simulink model "kh4_controller_v2"  (R2020a)
settings: Solver=ode15s  StartTime=0.0  StopTime=Inf  RelTol=1e-3
undefined symbols (not defined in the file or in its folder): Angular, Linear
libraries: robotlib x3, simulink x2, dspinverses x1
settings Model: Creator=FlightControlLab  LastModifiedBy=javier
settings SolverCC: SolverResetMethod=Robust
settings DataIOCC: ReturnWorkspaceOutputs=off
settings DebuggingCC: ArithmeticOperatorsInVariantConditions=warning
settings SFSimCC: SimUseLocalCustomCode=off  CustomCodeUndefinedFunction=UseInterfaceOnly
settings RTWCC: RTWUseLocalCustomCode=off

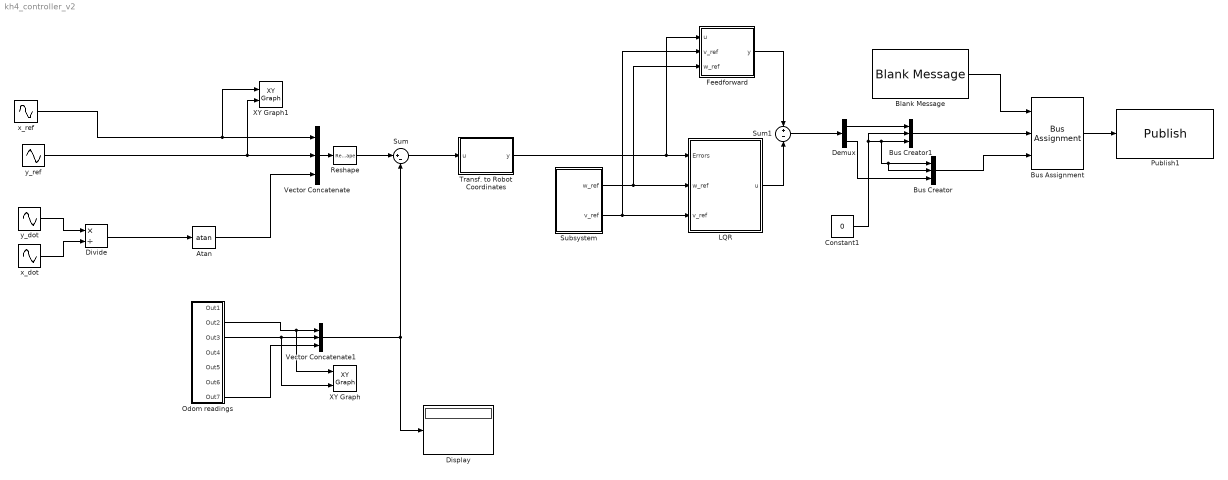
== system kh4_controller_v2 ==
  Atan : Trigonometry  Operator=atan
  Blank Message : robotlib/Blank Message  messageClass=Message  entityType=geometry_msgs/Twist  messageType=geometry_msgs/Twist  SampleTime=inf
  Bus Assignment : BusAssignment  AssignedSignals=Linear,Angular
  Bus Creator : BusCreator  Inputs=3
  Bus Creator1 : BusCreator  Inputs=3
  Constant1 : Constant  Value=0
  Demux : Demux  Outputs=2
  Display : Display
  Divide : Product  Inputs=*/
  Feedforward : MATLAB Function  TreatAsAtomicUnit=on
  LQR : Subsystem
  Odom readings : Subsystem
  Publish1 : robotlib/Publish  topicSource=Select from ROS network  topic=/kh4_diff_drive_controller/cmd_vel  messageType=geometry_msgs/Twist  messageQueueLength=105
  Reshape : Reshape  OutputDimensionality=Column vector (2-D)
  Subsystem : Subsystem
  Sum : Sum  Inputs=|+-
  Sum1 : Sum  Inputs=+-
  Transf. to Robot Coordinates : MATLAB Function  TreatAsAtomicUnit=on
  Vector Concatenate : Concatenate  NumInputs=3
  Vector Concatenate1 : Concatenate  NumInputs=3
  XY Graph : simulink/Sinks/XY Graph  xmin=-1  xmax=1  ymin=-1  ymax=1  st=-1
  XY Graph1 : simulink/Sinks/XY Graph  xmin=-1  xmax=1  ymin=-1  ymax=1  st=-1
  x_dot : Sin  Amplitude=0.3^2  Frequency=0.3  Phase=pi/2  SampleTime=0
  x_ref : Sin  Amplitude=0.3  Frequency=0.3  SampleTime=0
  y_dot : Sin  Amplitude=-0.3^2  Frequency=0.3  SampleTime=0
  y_ref : Sin  Amplitude=0.3  Bias=-0.3  Frequency=0.3  Phase=pi/2  SampleTime=0
  wires:
  x_dot/1 -> Divide/2
  Divide/1 -> Atan/1
  Sum/1 -> Transf. to Robot Coordinates/1(u)
  x_ref/1 -> XY Graph1/1, Vector Concatenate/1
  Vector Concatenate/1 -> Reshape/1
  y_ref/1 -> XY Graph1/2, Vector Concatenate/2
  Reshape/1 -> Sum/1
  Atan/1 -> Vector Concatenate/3
  Transf. to Robot Coordinates/1(y) -> LQR/1(Errors), Feedforward/1(u)
  Feedforward/1(y) -> Sum1/1
  Subsystem/2(v_ref) -> LQR/3(v_ref), Feedforward/2(v_ref)
  y_dot/1 -> Divide/1
  LQR/1(u) -> Sum1/2
  Subsystem/1(w_ref) -> LQR/2(w_ref), Feedforward/3(w_ref)
  Sum1/1 -> Demux/1
  Blank Message/1 -> Bus Assignment/1
  Bus Assignment/1 -> Publish1/1
  Constant1/1 -> Bus Creator1/2, Bus Creator/2, Bus Creator/1, Bus Creator1/3
  Demux/1 -> Bus Creator1/1
  Bus Creator/1 -> Bus Assignment/3
  Bus Creator1/1 -> Bus Assignment/2
  Demux/2 -> Bus Creator/3
  Odom readings/2(Out2) -> XY Graph/1, Vector Concatenate1/1
  Vector Concatenate1/1 -> Sum/2, Display/1
  Odom readings/7(Out7) -> Vector Concatenate1/3
  Odom readings/3(Out3) -> XY Graph/2, Vector Concatenate1/2

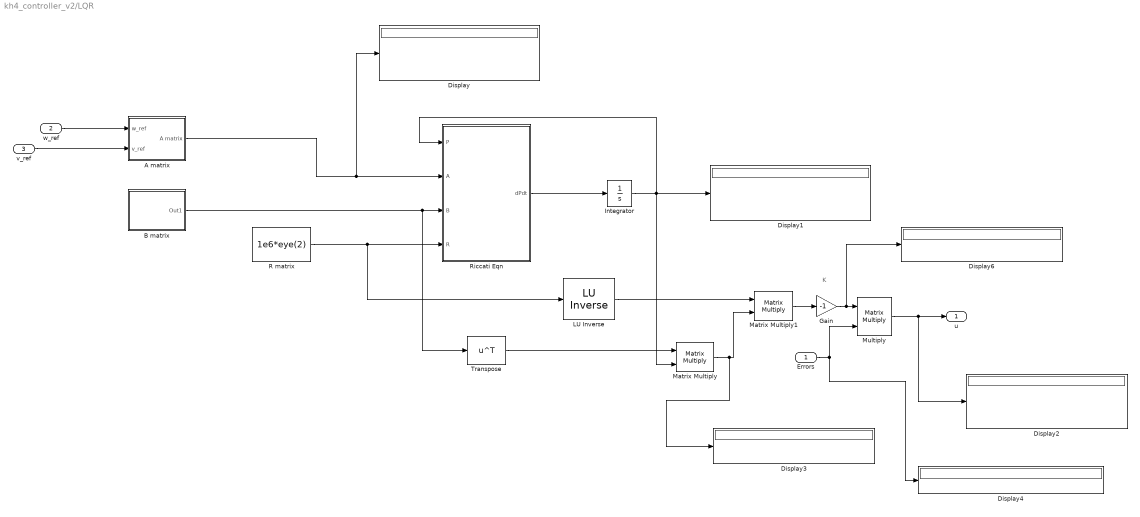
== system kh4_controller_v2/LQR ==
  note: K
  Errors : Inport
  w_ref : Inport  Port=2
  v_ref : Inport  Port=3
  " LU Inverse" : dspinverses/ LU Inverse
  A matrix : Subsystem
  B matrix : Subsystem
  Display{,1..4,6} (6 alike) : Display
  Gain : Gain  Gain=-1
  Integrator : Integrator
  Matrix Multiply : Product  Multiplication=Matrix(*)
  Matrix Multiply1 : Product  Multiplication=Matrix(*)
  Multiply : Product  Multiplication=Matrix(*)
  R matrix : Constant  Value=1e6*eye(2)  VectorParams1D=off
  Riccati Eqn : MATLAB Function  TreatAsAtomicUnit=on
  Transpose : Math  Operator=transpose  SignedPower=on  SaturateOnIntegerOverflow=on
  u : Outport  VectorParamsAs1DForOutWhenUnconnected=off
  wires:
  B matrix/1(Out1) -> Transpose/1, Riccati Eqn/3(B)
  R matrix/1 -> " LU Inverse"/1, Riccati Eqn/4(R)
  A matrix/1(A matrix) -> Display/1, Riccati Eqn/2(A)
  Multiply/1 -> Display2/1, u/1
  Integrator/1 -> Riccati Eqn/1(P), Display1/1, Matrix Multiply/2
  Matrix Multiply/1 -> Display3/1, Matrix Multiply1/2
  Transpose/1 -> Matrix Multiply/1
  Riccati Eqn/1(dPdt) -> Integrator/1
  w_ref/1 -> A matrix/1(w_ref)
  v_ref/1 -> A matrix/2(v_ref)
  Errors/1 -> Multiply/2, Display4/1
  " LU Inverse"/1 -> Matrix Multiply1/1
  Matrix Multiply1/1 -> Gain/1
  Gain/1 -> Display6/1, Multiply/1

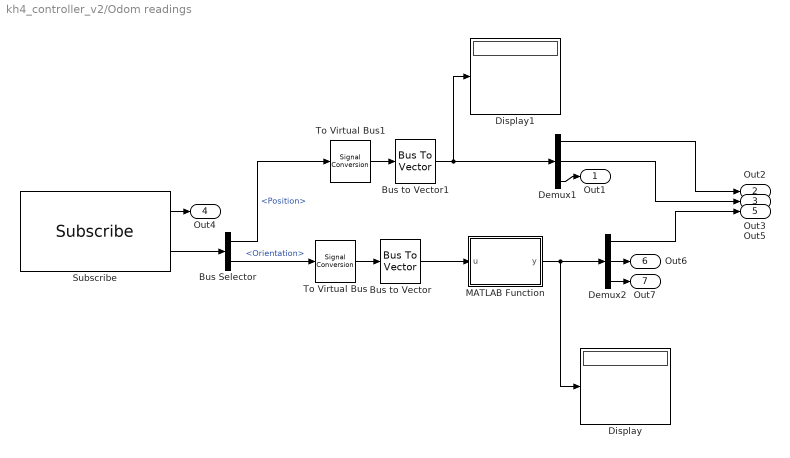
== system kh4_controller_v2/Odom readings ==
  Bus Selector : BusSelector  OutputSignals=Pose.Pose.Position,Pose.Pose.Orientation
  Bus to Vector : BusToVector
  Bus to Vector1 : BusToVector
  Demux1 : Demux  Outputs=3
  Demux2 : Demux  Outputs=3
  Display : Display
  Display1 : Display
  MATLAB Function : MATLAB Function  TreatAsAtomicUnit=on
  Subscribe : robotlib/Subscribe  topicSource=Select from ROS network  topic=/kh4_diff_drive_controller/odom  messageType=nav_msgs/Odometry  sampleTime=-1  messageQueueLength=1
  To Virtual Bus : SignalConversion  ConversionOutput=Virtual bus  OverrideOpt=off
  To Virtual Bus1 : SignalConversion  ConversionOutput=Virtual bus  OverrideOpt=off
  Out1 : Outport
  Out2 : Outport  Port=2
  Out3 : Outport  Port=3
  Out4 : Outport  Port=4
  Out5 : Outport  Port=5
  Out6 : Outport  Port=6
  Out7 : Outport  Port=7
  wires:
  Demux2/2 -> Out6/1
  Bus Selector/1 -> To Virtual Bus1/1  "<Position>"
  Demux1/1 -> Out2/1
  Demux1/2 -> Out3/1
  MATLAB Function/1(y) -> Demux2/1, Display/1
  Demux2/1 -> Out5/1
  Bus to Vector/1 -> MATLAB Function/1(u)
  Subscribe/1 -> Out4/1
  Demux2/3 -> Out7/1
  Bus to Vector1/1 -> Demux1/1, Display1/1
  Bus Selector/2 -> To Virtual Bus/1  "<Orientation>"
  Demux1/3 -> Out1/1
  To Virtual Bus/1 -> Bus to Vector/1
  Subscribe/2 -> Bus Selector/1
  To Virtual Bus1/1 -> Bus to Vector1/1

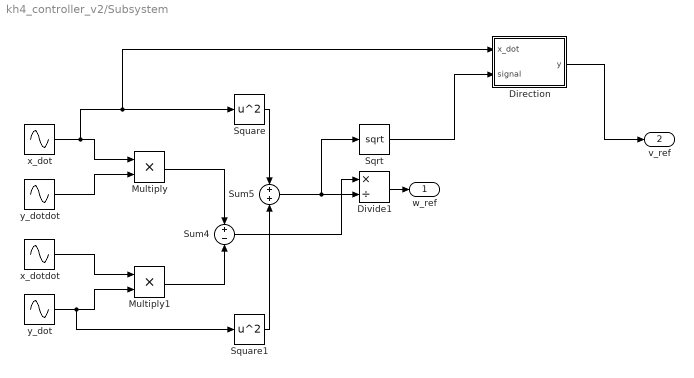
== system kh4_controller_v2/Subsystem ==
  Direction : MATLAB Function  TreatAsAtomicUnit=on
  Divide1 : Product  Inputs=*/
  Multiply : Product
  Multiply1 : Product
  Sqrt : Sqrt  SaturateOnIntegerOverflow=on
  Square : Math  Operator=square  SignedPower=on  SaturateOnIntegerOverflow=on
  Square1 : Math  Operator=square  SignedPower=on  SaturateOnIntegerOverflow=on
  Sum4 : Sum  Inputs=+-
  Sum5 : Sum
  x_dot : Sin  Amplitude=0.3^2  Frequency=0.3  Phase=pi/2  SampleTime=0
  x_dotdot : Sin  Amplitude=-0.3^3  Frequency=0.3  SampleTime=0
  y_dot : Sin  Amplitude=-0.3^2  Frequency=0.3  SampleTime=0
  y_dotdot : Sin  Amplitude=-0.3^3  Frequency=0.3  Phase=pi/2  SampleTime=0
  w_ref : Outport  VectorParamsAs1DForOutWhenUnconnected=off
  v_ref : Outport  Port=2  VectorParamsAs1DForOutWhenUnconnected=off
  wires:
  x_dot/1 -> Direction/1(x_dot), Square/1, Multiply/1
  Divide1/1 -> w_ref/1
  x_dotdot/1 -> Multiply1/1
  Sum5/1 -> Divide1/2, Sqrt/1
  Square/1 -> Sum5/1
  Sum4/1 -> Divide1/1
  y_dot/1 -> Square1/1, Multiply1/2
  y_dotdot/1 -> Multiply/2
  Multiply1/1 -> Sum4/2
  Square1/1 -> Sum5/2
  Multiply/1 -> Sum4/1
  Sqrt/1 -> Direction/2(signal)
  Direction/1(y) -> v_ref/1

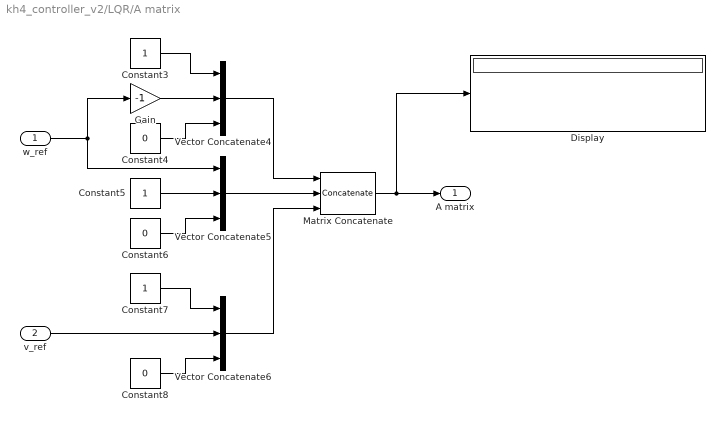
== system kh4_controller_v2/LQR/A matrix ==
  w_ref : Inport
  v_ref : Inport  Port=2
  Constant3 : Constant
  Constant4 : Constant  Value=0
  Constant5 : Constant
  Constant6 : Constant  Value=0
  Constant7 : Constant
  Constant8 : Constant  Value=0
  Display : Display
  Gain : Gain  Gain=-1
  Matrix Concatenate : Concatenate  NumInputs=3  Mode=Multidimensional array  ConcatenateDimension=2
  Vector Concatenate4 : Concatenate  NumInputs=3
  Vector Concatenate5 : Concatenate  NumInputs=3
  Vector Concatenate6 : Concatenate  NumInputs=3
  A matrix : Outport  VectorParamsAs1DForOutWhenUnconnected=off
  wires:
  w_ref/1 -> Gain/1, Vector Concatenate5/1
  Gain/1 -> Vector Concatenate4/2
  Constant6/1 -> Vector Concatenate5/3
  Vector Concatenate6/1 -> Matrix Concatenate/3
  Constant4/1 -> Vector Concatenate4/3
  v_ref/1 -> Vector Concatenate6/2
  Constant7/1 -> Vector Concatenate6/1
  Vector Concatenate5/1 -> Matrix Concatenate/2
  Constant8/1 -> Vector Concatenate6/3
  Constant3/1 -> Vector Concatenate4/1
  Constant5/1 -> Vector Concatenate5/2
  Vector Concatenate4/1 -> Matrix Concatenate/1
  Matrix Concatenate/1 -> Display/1, A matrix/1

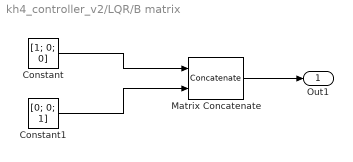
== system kh4_controller_v2/LQR/B matrix ==
  Constant : Constant  Value=[1; 0; 0]  VectorParams1D=off
  Constant1 : Constant  Value=[0; 0; 1]  VectorParams1D=off
  Matrix Concatenate : Concatenate  Mode=Multidimensional array  ConcatenateDimension=2
  Out1 : Outport  VectorParamsAs1DForOutWhenUnconnected=off
  wires:
  Constant/1 -> Matrix Concatenate/1
  Matrix Concatenate/1 -> Out1/1
  Constant1/1 -> Matrix Concatenate/2

== matlab function kh4_controller_v2/Subsystem/Direction ==
  data: x_dot input; y output; signal input
function y = fcn(x_dot, signal)
if x_dot < 0
    y = -signal;
else
    y = signal;
end
end

== matlab function kh4_controller_v2/Transf. to Robot Coordinates ==
  data: u input size=[3,1]; y output size=[3,1]
function y = fcn(u)

theta = u(3);
A = [cos(theta), sin(theta), 0;
    -sin(theta), cos(theta), 0;
    0, 0, 1];

y = A*u;

== matlab function kh4_controller_v2/Feedforward ==
  data: u input size=[3,1]; y output size=[2,1]; v_ref input size=1; w_ref input size=1
function y = fcn(u, v_ref, w_ref)

    e3 = u(3);
    
    y = [cos(e3)*v_ref;
        w_ref];

== matlab function kh4_controller_v2/Odom readings/MATLAB Function ==
  data: u input; y output
function y = fcn(u)

y = quat2eul(u');

== matlab function kh4_controller_v2/LQR/Riccati Eqn ==
  data: dPdt output size=[3,3]; P input size=[3,3]; A input size=[3,3]; B input size=[3,2]; R input size=[2,2]
function dPdt = mRiccati(P,A,B,R)

% A = rand(3,3);
% B = rand(3,2);
Q = diag([1 1 10]);
% R = 1e-4*diag([1 1]);
% P = rand(3,3);


% Continuous Riccati differential equation
dPdt = -(A'*P + P*A - (P*B)*pinv(R)*(B'*P) + Q);
